simulink model "EncoderControl"  (R2021a)
settings: Solver=FixedStepAuto  StartTime=0.0  StopTime=100.0  FixedStep=0.001  RelTol=1e-3  EnableMultiTasking=on
libraries: arduinolib x2, simulink x1
settings Model: SILPILModeSetting=veronly  ExtModeTrigDuration=2  Creator=Samuel  LastModifiedBy=drak0
settings OptimizationCC: EnhancedBackFolding=on  PassReuseOutputArgsAs=Individual arguments  ZeroExternalMemoryAtStartup=off  ZeroInternalMemoryAtStartup=off  MaxStackSize=64  OptimizeBlockOrder=speed  DifferentSizesBufferReuse=on  OptimizationCustomize=off  EfficientTunableParamExpr=on
settings DebuggingCC: ParameterTunabilityLossMsg=error
settings HardwareCC: ProdBitPerInt=16  ProdBitPerPointer=16  ProdBitPerSizeT=16  ProdBitPerPtrDiffT=16  ProdLargestAtomicFloat=None  ProdWordSize=8  ProdHWDeviceType=Atmel->AVR  UseEmbeddedCoderFeatures=off  UseSimulinkCoderFeatures=off
settings SFSimCC: MATLABDynamicMemAlloc=off
settings RTWCC: SystemTargetFile=ert.tlc  HardwareBoard=Arduino Mega 2560  TemplateMakefile=ert_default_tmf  Toolchain=Arduino AVR  BuildConfiguration=Faster Runs
settings CodeAppCC: ForceParamTrailComments=on  IgnoreCustomStorageClasses=off  OperatorAnnotations=on  SimulinkDataObjDesc=on  SFDataObjDesc=on  InsertBlockDesc=on
settings ERTTargetCC: SupportContinuousTime=on  SupportNonInlinedSFcns=on  SupportVariableSizeSignals=on  ExtModeStaticAllocSize=2048

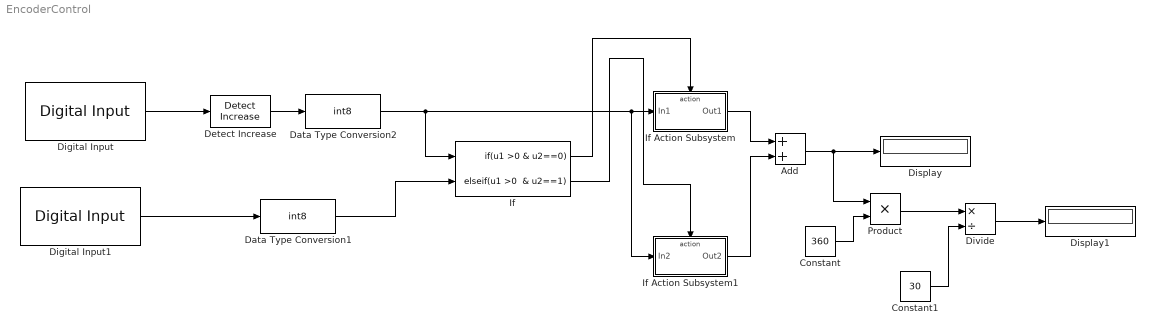
== system EncoderControl ==
  Add : Sum
  Constant : Constant  Value=360
  Constant1 : Constant  Value=30
  Data Type Conversion1 : DataTypeConversion  OutDataTypeStr=int8
  Data Type Conversion2 : DataTypeConversion  OutDataTypeStr=int8
  Detect Increase : simulink/Logic and Bit Operations/Detect Increase  vinit=0.0  OutDataTypeStr=boolean
  Digital Input : arduinolib/Digital Input  pinNumber=2  mode=Default  Direction=input  SampleTime=-1  blockPlatform=arduino
  Digital Input1 : arduinolib/Digital Input  pinNumber=3  mode=Default  Direction=input  SampleTime=-1  blockPlatform=arduino
  Display : Display
  Display1 : Display
  Divide : Product  Inputs=*/
  If : If  NumInputs=2  IfExpression=u1 >0 & u2==0  ElseIfExpressions="u1 >0  & u2==1"  ShowElse=off
  If Action Subsystem : Subsystem  TreatAsAtomicUnit=on
  If Action Subsystem1 : Subsystem  TreatAsAtomicUnit=on
  Product : Product
  wires:
  Digital Input/1 -> Detect Increase/1
  Data Type Conversion1/1 -> If/2
  If/2 -> If Action Subsystem1/Action
  If/1 -> If Action Subsystem/Action
  If Action Subsystem/1(Out1) -> Add/1
  If Action Subsystem1/1(Out2) -> Add/2
  Add/1 -> Product/1, Display/1
  Constant/1 -> Product/2
  Product/1 -> Divide/1
  Constant1/1 -> Divide/2
  Divide/1 -> Display1/1
  Detect Increase/1 -> Data Type Conversion2/1
  Data Type Conversion2/1 -> If Action Subsystem1/1(In2), If Action Subsystem/1(In1), If/1
  Digital Input1/1 -> Data Type Conversion1/1

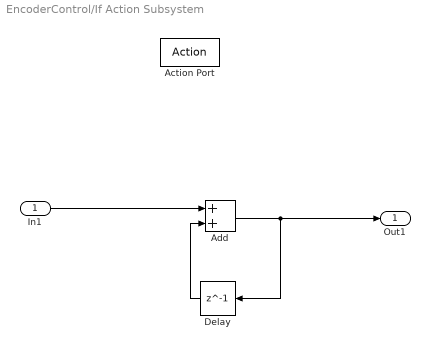
== system EncoderControl/If Action Subsystem ==
  In1 : Inport
  Action Port : ActionPort  ActionPortLabel=if(u1 >0 & u2==0)
  Add : Sum
  Delay : Delay  DelayLength=1  InitialCondition=0
  Out1 : Outport
  wires:
  In1/1 -> Add/1
  Add/1 -> Delay/1, Out1/1
  Delay/1 -> Add/2

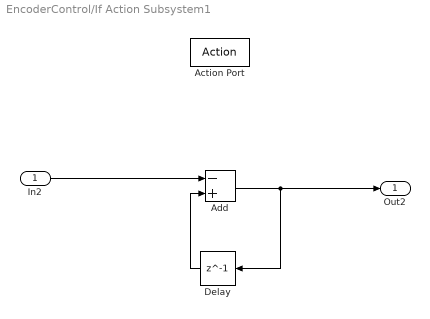
== system EncoderControl/If Action Subsystem1 ==
  In2 : Inport
  Action Port : ActionPort  ActionPortLabel="elseif( u1 >0  & u2==1)"
  Add : Sum  Inputs=-+
  Delay : Delay  DelayLength=1  InitialCondition=0
  Out2 : Outport
  wires:
  In2/1 -> Add/1
  Delay/1 -> Add/2
  Add/1 -> Delay/1, Out2/1
